simulink model "lab12_2"  (R2017a)
settings: Solver=VariableStepAuto  StartTime=0.0  StopTime=1  RelTol=1e-3
settings Model: Creator=Peter  LastModifiedBy=Peter

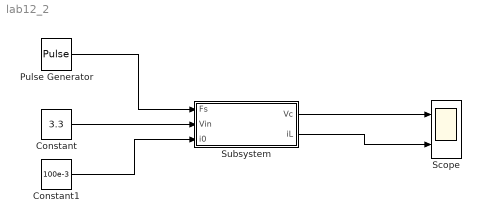
== system lab12_2 ==
  Constant : Constant  Value=3.3
  Constant1 : Constant  Value=100e-3
  Pulse Generator : DiscretePulseGenerator  PulseType=Time based  Period=1*10^-6  PulseWidth=36.45
  Scope : Scope  NumInputPorts=2
  Subsystem : Subsystem
  wires:
  Subsystem/1(Vc) -> Scope/1
  Constant/1 -> Subsystem/2(Vin)
  Constant1/1 -> Subsystem/3(i0)
  Pulse Generator/1 -> Subsystem/1(Fs)
  Subsystem/2(iL) -> Scope/2

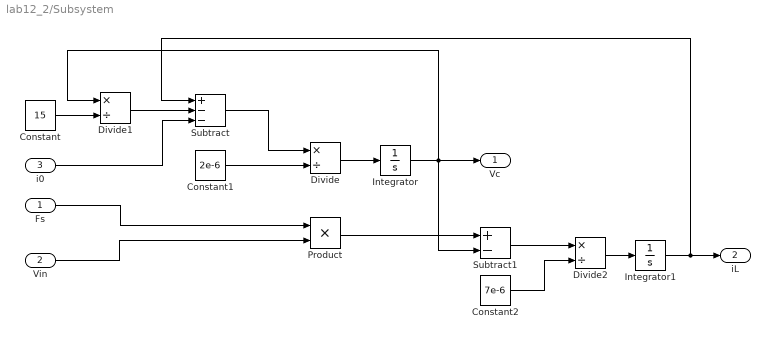
== system lab12_2/Subsystem ==
  Fs : Inport
  Vin : Inport  Port=2
  i0 : Inport  Port=3
  Constant : Constant  Value=15
  Constant1 : Constant  Value=2e-6
  Constant2 : Constant  Value=7e-6
  Divide : Product  Inputs=*/
  Divide1 : Product  Inputs=*/
  Divide2 : Product  Inputs=*/
  Integrator : Integrator
  Integrator1 : Integrator
  Product : Product
  Subtract : Sum  Inputs=+--
  Subtract1 : Sum  Inputs=+-
  Vc : Outport
  iL : Outport  Port=2
  wires:
  Divide/1 -> Integrator/1
  Integrator/1 -> Subtract1/2, Divide1/1, Vc/1
  Divide1/1 -> Subtract/2
  i0/1 -> Subtract/3
  Subtract/1 -> Divide/1
  Fs/1 -> Product/1
  Vin/1 -> Product/2
  Product/1 -> Subtract1/1
  Subtract1/1 -> Divide2/1
  Divide2/1 -> Integrator1/1
  Integrator1/1 -> Subtract/1, iL/1
  Constant/1 -> Divide1/2
  Constant1/1 -> Divide/2
  Constant2/1 -> Divide2/2
